simulink model "TORQUECONTROL"  (R2024b)
settings: Solver=FixedStepAuto  StartTime=0.0  StopTime=10.0  RelTol=1e-3  EnableMultiTasking=on
settings Model: DataDictionary=Master_Dictionary.sldd  EnableAccessToBaseWorkspace=off  Creator=torni  LastModifiedBy=Will
settings OptimizationCC: DefaultParameterBehavior=Inlined  EnhancedBackFolding=on  PassReuseOutputArgsAs=Individual arguments  ZeroExternalMemoryAtStartup=off  ZeroInternalMemoryAtStartup=off  MaxStackSize=8192  OptimizeBlockOrder=speed  DifferentSizesBufferReuse=on  OptimizationCustomize=off  EfficientTunableParamExpr=on
settings DebuggingCC: ParameterTunabilityLossMsg=error
settings HardwareCC: ProdBitPerPointer=32  ProdBitPerSizeT=32  ProdBitPerPtrDiffT=32  ProdLargestAtomicInteger=Long  ProdLargestAtomicFloat=Double  ProdWordSize=32  ProdLongLongMode=on  ProdHWDeviceType=ARM Compatible->ARM Cortex-M
settings SFSimCC: MATLABDynamicMemAlloc=off
settings RTWCC: Description=Embedded Coder  SystemTargetFile=ert.tlc  HardwareBoard=STM32H7xx Based (Single-core)  TemplateMakefile=ert_default_tmf  Toolchain=GNU Tools for ARM Embedded Processors
settings CodeAppCC: ForceParamTrailComments=on  IgnoreCustomStorageClasses=off  OperatorAnnotations=on  SimulinkDataObjDesc=on  SFDataObjDesc=on  InsertBlockDesc=on
settings ERTTargetCC: TargetLangStandard=C99 (ISO)  CodeReplacementLibrary=ARM Cortex-M  ExtModeTransport=3  ExtModeStaticAlloc=on  ExtModeStaticAllocSize=2048  ExtModeMexFile=ext_xcp  ExtModeIntrfLevel=Level2 - Open

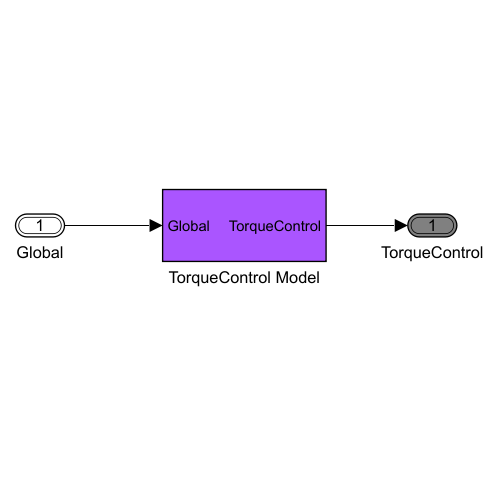
[thumbnail: Simulink's stored preview of the top-level diagram]
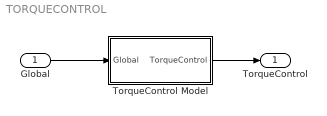
== system TORQUECONTROL ==
  "Global " : Inport  OutDataTypeStr=Bus: Global
  "TorqueControl Model " : Subsystem
  TorqueControl : Outport  OutDataTypeStr=Bus: TorqueControl  VectorParamsAs1DForOutWhenUnconnected=off
  wires:
  "Global "/1 -> "TorqueControl Model "/1(Global)
  "TorqueControl Model "/1(TorqueControl) -> TorqueControl/1

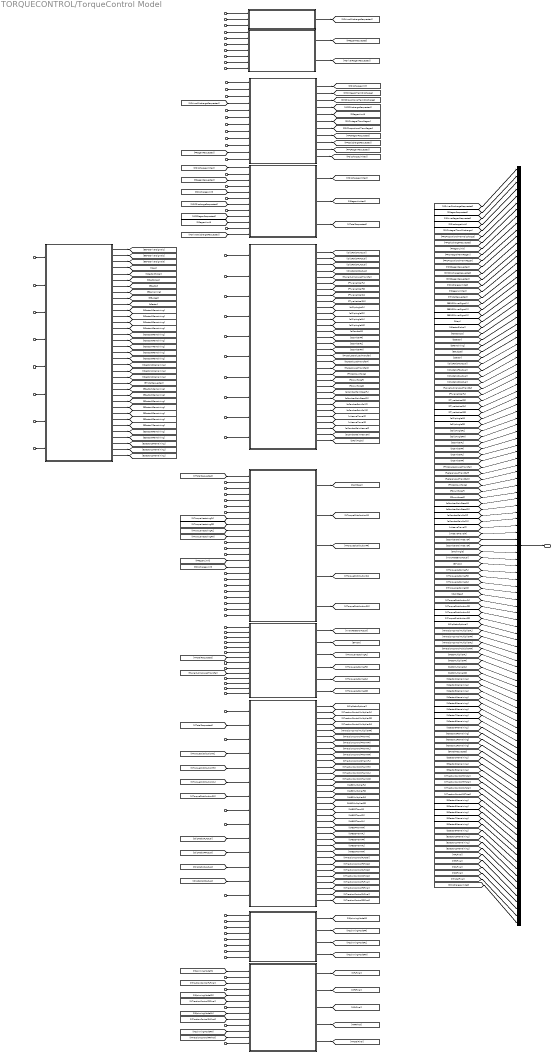
== system TORQUECONTROL/TorqueControl Model  ==
  note: Final output
  note: Distribution
  note: Energy & Vehicle State
  note: Total Torque Request
  note: Driver Requests
  note: Stages of Torque Control
      | 1. Driver Request
      | 2. Power Controller
      | 3. Total Torque Request
      | 4. Torque Distribution / Torque Vectoring
      | 5. Traction Control
      | 6. Spinning Mode Selection
  In Bus Element70 : Inport  PortName=Global  Element=InverterSignals.InverterRLSignals.nMotorRL
  In Bus Element74 : Inport  PortName=Global  Element=InverterSignals.InverterRLSignals.VDCInvRL
  In Bus Element : Inport  PortName=Global  Element=InverterSignals.InverterFLSignals.nMotorFL
  In Bus Element2 : Inport  PortName=Global  Element=InverterSignals.InverterRRSignals.nMotorRR
  In Bus Element3 : Inport  PortName=Global  Element=InverterSignals.InverterFRSignals.nMotorFR
  In Bus Element4 : Inport  PortName=Global  Element=Systems.pBrakeMax
  In Bus Element17 : Inport  PortName=Global  Element=Systems.pBrakeMax
  In Bus Element49 : Inport  PortName=Global  Element=Systems.pBrakeMax
  In Bus Element6 : Inport  PortName=Global  Element=Systems.BSpinningModeOn
  In Bus Element21 : Inport  PortName=Global  Element=Systems.BSpinningModeOn
  In Bus Element{7,16,37,48,57,62,79} (7 alike) : Inport  PortName=Global  Element=Systems.rThrottlePedal
  In Bus Element8 : Inport  PortName=Global  Element=Systems.NTCKdSelector
  In Bus Element{9,18,38..39,59,64,71,78} (8 alike) : Inport  PortName=Global  Element=Systems.vChassis
  In Bus Element10 : Inport  PortName=Global  Element=Systems.BTCOn
  In Bus Element11 : Inport  PortName=Global  Element=Systems.rGrip
  In Bus Element12 : Inport  PortName=Global  Element=Systems.rSteeringAngle
  In Bus Element14 : Inport  PortName=Global  Element=Systems.rTVMultiplier
  In Bus Element15 : Inport  PortName=Global  Element=Systems.BTVOn
  In Bus Element32 : Inport  PortName=Global  Element=Systems.BTVOn
  In Bus Element19 : Inport  PortName=Global  Element=Systems.aSteeringAngle
  In Bus Element1 : Inport  PortName=Global  Element=Systems.aSteeringAngle
  In Bus Element30 : Inport  PortName=Global  Element=Systems.rTorqueSplit
  In Bus Element31 : Inport  PortName=Global  Element=Systems.rEngineBrakingSplit
  In Bus Element33 : Inport  PortName=Global  Element=Systems.PEngineBraking
  In Bus Element34 : Inport  PortName=Global  Element=Systems.BInverterErrorFront
  In Bus Element35 : Inport  PortName=Global  Element=Systems.BInverterErrorRear
  In Bus Element{36,50,53,60,75} (5 alike) : Inport  PortName=Global  Element=Systems.rRegenPaddle
  In Bus Element51 : Inport  PortName=Global  Element=Systems.PActual
  In Bus Element58 : Inport  PortName=Global  Element=Systems.PActual
  In Bus Element63 : Inport  PortName=Global  Element=Systems.PActual
  In Bus Element52 : Inport  PortName=Global  Element=Systems.BEMSOn
  In Bus Element54 : Inport  PortName=Global  Element=Systems.sChassis
  In Bus Element55 : Inport  PortName=Global  Element=Systems.EOffset
  In Bus Element56 : Inport  PortName=Global  Element=Systems.rSOE
  In Bus Element67 : Inport  PortName=Global  Element=Systems.PRegenMax
  In Bus Element61 : Inport  PortName=Global  Element=Systems.PRegenMax
  In Bus Element68 : Inport  PortName=Global  Element=Systems.PDischargeMax
  In Bus Element69 : Inport  PortName=Global  Element=Systems.NPCKpSelector
  In Bus Element76 : Inport  PortName=Global  Element=Systems.MRegenMax
  In Bus Element77 : Inport  PortName=Global  Element=Systems.NThrottleMap
  In Bus Element81 : Inport  PortName=Global  Element=Systems.MMotorMaxFL
  In Bus Element86 : Inport  PortName=Global  Element=Systems.MMotorMaxFL
  In Bus Element83 : Inport  PortName=Global  Element=Systems.MMotorMaxFR
  In Bus Element87 : Inport  PortName=Global  Element=Systems.MMotorMaxFR
  In Bus Element84 : Inport  PortName=Global  Element=Systems.MMotorMaxRL
  In Bus Element88 : Inport  PortName=Global  Element=Systems.MMotorMaxRL
  In Bus Element85 : Inport  PortName=Global  Element=Systems.MMotorMaxRR
  In Bus Element89 : Inport  PortName=Global  Element=Systems.MMotorMaxRR
  In Bus Element5 : Inport  PortName=Global  Element=Stateflow.BReadyToDrive
  In Bus Element13 : Inport  PortName=Global  Element=GPSIMUSignals.nYawRateIMU
  In Bus Element40 : Inport  PortName=Global  Element=GPSIMUSignals.nYawRateIMU
  In Bus Element20 : Inport  PortName=Global  Element=GPSIMUSignals.gLongitudinalIMU
  In Bus Element42 : Inport  PortName=Global  Element=GPSIMUSignals.gLongitudinalIMU
  In Bus Element43 : Inport  PortName=Global  Element=GPSIMUSignals.gLateralIMU
  In Bus Element41 : Inport  PortName=Global  Element=GPSIMUSignals.vLateralIMU
  In Bus Element22 : Inport  PortName=Global  Element=Limitations.rSpeedRegenDerateFL
  In Bus Element23 : Inport  PortName=Global  Element=Limitations.rSpeedRegenDerateFR
  In Bus Element24 : Inport  PortName=Global  Element=Limitations.rSpeedRegenDerateRL
  In Bus Element25 : Inport  PortName=Global  Element=Limitations.rSpeedRegenDerateRR
  In Bus Element26 : Inport  PortName=Global  Element=Limitations.PTSTemperatureDerateRR
  In Bus Element27 : Inport  PortName=Global  Element=Limitations.PTSTemperatureDerateRL
  In Bus Element28 : Inport  PortName=Global  Element=Limitations.PTSTemperatureDerateFR
  In Bus Element29 : Inport  PortName=Global  Element=Limitations.PTSTemperatureDerateFL
  In Bus Element65 : Inport  PortName=Global  Element=Limitations.PRegenDerate
  In Bus Element80 : Inport  PortName=Global  Element=Limitations.PRegenDerate
  In Bus Element66 : Inport  PortName=Global  Element=Limitations.PDischargeDerate
  In Bus Element72 : Inport  PortName=Global  Element=Limitations.BDischargeAllowed
  In Bus Element82 : Inport  PortName=Global  Element=Limitations.BDischargeAllowed
  In Bus Element44 : Inport  PortName=Global  Element=WheelSpeeds.vWheelRR
  In Bus Element45 : Inport  PortName=Global  Element=WheelSpeeds.vWheelRL
  In Bus Element46 : Inport  PortName=Global  Element=WheelSpeeds.vWheelFR
  In Bus Element47 : Inport  PortName=Global  Element=WheelSpeeds.vWheelFL
  In Bus Element73 : Inport  PortName=Global  Element=BMSSignals.IIVTS
  Bus Creator1 : BusCreator  Inputs=113  OutDataTypeStr=Bus: TorqueControl
  Model : ModelReference  ModelNameDialog=MDriverRegenRequested.slx  SimulationMode=Normal  ModelReferenceVersion=13.6
  Model1 : ModelReference  ModelNameDialog=StateEstimation.slx  SimulationMode=Normal  ModelReferenceVersion=13.6
  Model10 : ModelReference  ModelNameDialog=MFinal.slx  SimulationMode=Normal  ModelReferenceVersion=13.6
  Model2 : ModelReference  ModelNameDialog=MDriverDischargeRequested.slx  SimulationMode=Normal  ModelReferenceVersion=13.6
  Model3 : ModelReference  ModelNameDialog=PowerController.slx  SimulationMode=Normal  ModelReferenceVersion=13.6
  Model4 : ModelReference  ModelNameDialog=MTotalRequested.slx  SimulationMode=Normal  ModelReferenceVersion=13.6
  Model5 : ModelReference  ModelNameDialog=EMS.slx  SimulationMode=Normal  ModelReferenceVersion=13.6
  Model6 : ModelReference  ModelNameDialog=TorqueVectoring.slx  SimulationMode=Normal  ModelReferenceVersion=13.6
  Model7 : ModelReference  ModelNameDialog=TorqueDistribution.slx  SimulationMode=Normal  ModelReferenceVersion=13.6
  Model8 : ModelReference  ModelNameDialog=TractionControl.slx  SimulationMode=Normal  ModelReferenceVersion=13.6
  Model9 : ModelReference  ModelNameDialog=SpinningMode.slx  SimulationMode=Normal  ModelReferenceVersion=13.6
  TorqueControl : Outport  OutDataTypeStr=Bus: TorqueControl  VectorParamsAs1DForOutWhenUnconnected=off
  wires:
  Model7/1 -> [rSplitRear]
  Model7/2 -> [MTorqueDistributionFL]
  Model7/3 -> [MTorqueDistributionFR]
  Model7/4 -> [MTorqueDistributionRL]
  Model7/5 -> [MTorqueDistributionRR]
  Model9/1 -> [MSpinningModeFL]
  Model9/2 -> [MSpinningModeFR]
  Model9/3 -> [MSpinningModeRL]
  Model9/4 -> [MSpinningModeRR]
  Bus Creator1/1 -> TorqueControl/1
  [MDriverDischargeRequested] -> Bus Creator1/1  "MDriverDischargeRequested"
  [MDriverRegenRequested] -> Bus Creator1/3  "MDriverRegenRequested"
  [MTotalRequested] -> Model7/1
  Model4/1 -> [MDischargeLimited]
  Model4/2 -> [MRegenLimited]
  Model4/3 -> [MTotalRequested]
  [PDischargeLimit] -> Model4/5
  [PRegenRequested] -> Model4/3
  [PDischargeLimited] -> Model4/1
  [MDischargeLimited] -> Bus Creator1/14  "MDischargeLimited"
  [MRegenLimited] -> Bus Creator1/15  "MRegenLimited"
  Model1/1 -> [rSlipRatioFLActual]
  Model1/2 -> [rSlipRatioFRActual]
  Model1/3 -> [rSlipRatioRLActual]
  Model1/4 -> [rSlipRatioRRActual]
  Model1/5 -> [FLongitudinalLoadTransfer]
  Model1/6 -> [FTyreVerticalFL]
  Model1/7 -> [FTyreVerticalFR]
  Model1/8 -> [FTyreVerticalRL]
  Model1/9 -> [FTyreVerticalRR]
  Model1/10 -> [aSlipAngleFL]
  Model1/11 -> [aSlipAngleFR]
  Model1/12 -> [aSlipAngleRL]
  Model1/13 -> [aSlipAngleRR]
  Model1/14 -> [aCamberFL]
  Model1/15 -> [aCamberFR]
  Model1/16 -> [aCamberRL]
  Model1/17 -> [aCamberRR]
  Model1/18 -> [FTotalLateralLoadTransfer]
  Model1/19 -> [FLateralLoadTransferF]
  Model1/20 -> [FLateralLoadTransferR]
  Model1/21 -> [FTotalDownforce]
  Model1/22 -> [FDownforceF]
  Model1/23 -> [FDownforceR]
  Model1/24 -> [aCamberGainSteerFL]
  Model1/25 -> [aCamberGainSteerFR]
  Model1/26 -> [aCamberGainRollF]
  Model1/27 -> [aCamberGainRollR]
  Model1/28 -> [xHeaveTravelF]
  Model1/29 -> [xHeaveTravelR]
  Model1/30 -> [aCamberGainHeaveF]
  Model1/31 -> [aCamberGainHeaveR]
  Model1/32 -> [aRollAngle]
  In Bus Element39/1 -> Model1/1
  In Bus Element47/1 -> Model1/2
  Model2/1 -> [MDriverDischargeRequested]
  Model10/1 -> [MFLFinal]
  Model10/2 -> [MFRFinal]
  Model10/3 -> [MRLFinal]
  Model10/4 -> [MRRFinal]
  Model10/5 -> [MTotalFinal]
  [MTractionControlFLFinal] -> Model10/3
  [MTractionControlFRFinal] -> Model10/6
  [MTractionControlRLFinal] -> Model10/9
  [MSpinningModeFL] -> Model10/1
  [MSpinningModeFR] -> Model10/5
  [MSpinningModeRL] -> Model10/8
  [MTorqueDistributionFL] -> Model8/4
  [MTorqueDistributionFR] -> Model8/5
  [MTorqueDistributionRL] -> Model8/6
  [MTorqueDistributionRR] -> Model8/7
  Model8/33 -> [MTractionControlRRFinal]
  Model8/32 -> [MTractionControlRLFinal]
  Model8/31 -> [MTractionControlFRFinal]
  Model8/30 -> [MTractionControlFLFinal]
  Model8/29 -> [MTractionControlRRTotal]
  Model8/28 -> [MTractionControlRLTotal]
  Model8/27 -> [MTractionControlFRTotal]
  Model8/26 -> [MTractionControlFLTotal]
  Model8/14 -> [NABSMultiplierFL]
  Model8/15 -> [NABSMultiplierFR]
  Model8/16 -> [NABSMultiplierRL]
  Model8/17 -> [NABSMultiplierRR]
  [MTotalRequested] -> Model8/2
  Model8/1 -> [rSlipRatioOptimal]
  Model8/2 -> [NTractionControlMultiplierFL]
  Model8/3 -> [NTractionControlMultiplierFR]
  Model8/4 -> [NTractionControlMultiplierRL]
  Model8/5 -> [NTractionControlMultiplierRR]
  Model8/6 -> [NTractionControlPTermFL]
  Model8/7 -> [NTractionControlPTermFR]
  Model8/8 -> [NTractionControlPTermRL]
  Model8/9 -> [NTractionControlPTermRR]
  Model8/13 -> [NTractionControlDTermRR]
  Model8/12 -> [NTractionControlDTermRL]
  Model8/10 -> [NTractionControlDTermFL]
  Model8/11 -> [NTractionControlDTermFR]
  Model8/18 -> [NABSPTermFL]
  Model8/19 -> [NABSPTermFR]
  Model8/20 -> [NABSPTermRL]
  Model8/21 -> [NABSPTermRR]
  Model8/22 -> [NABSDTermFL]
  Model8/23 -> [NABSDTermFR]
  Model8/24 -> [NABSDTermRL]
  Model8/25 -> [NABSDTermRR]
  [MDriverDischargeRequested] -> Model3/4
  Model/1 -> [PRegenRequested]
  [PRegenRequested] -> Bus Creator1/2  "PRegenRequested"
  [MTorqueVectoringFL] -> Model7/8
  [MTorqueVectoringRR] -> Model7/11
  [MTorqueVectoringRL] -> Model7/10
  [MTorqueVectoringFR] -> Model7/9
  Model5/1 -> [BEMSDriverSignal1]
  Model5/2 -> [BEMSDriverSignal2]
  Model5/4 -> [NLap]
  Model5/3 -> [BEMSDriverSignal3]
  Model3/10 -> [PPCRegenRequested]
  Model3/9 -> [PPCDischargeRequested]
  Model3/8 -> [MPCRegenRequested]
  Model3/7 -> [PPCProportionalTermRegen]
  Model3/6 -> [PPCIntegralTermRegen]
  Model3/5 -> [PRegenLimit]
  Model3/4 -> [MPCDischargeRequested]
  Model3/3 -> [PPCProportionalTermDischarge]
  Model3/2 -> [PPCIntegralTermDischarge]
  Model3/1 -> [PDischargeLimit]
  [PDischargeLimit] -> Bus Creator1/4  "PDischargeLimit"
  [PPCIntegralTermDischarge] -> Bus Creator1/5  "PPCIntegralTermDischarge"
  [PPCProportionalTermDischarge] -> Bus Creator1/6  "PPCProportionalTermDischarge"
  [MPCDischargeRequested] -> Bus Creator1/7  "MPCDischargeRequested"
  [PRegenLimit] -> Bus Creator1/8  "PRegenLimit"
  [PPCIntegralTermRegen] -> Bus Creator1/9  "PPCIntegralTermRegen"
  [PPCProportionalTermRegen] -> Bus Creator1/10  "PPCProportionalTermRegen"
  [MPCRegenRequested] -> Bus Creator1/11  "MPCRegenRequested"
  [PPCDischargeRequested] -> Bus Creator1/12  "PPCDischargeRequested"
  [PPCRegenRequested] -> Bus Creator1/13  "PPCRegenRequested"
  [PRegenRequested] -> Model3/11
  Model3/11 -> [PDischargeLimited]
  Model5/5 -> [NSectorGlobal]
  Model5/6 -> [NSectorLap]
  Model5/7 -> [ESector]
  Model5/8 -> [ERemaining]
  Model5/9 -> [EBudget]
  Model5/10 -> [sSector]
  In Bus Element73/1 -> Model/6
  [MPCDischargeRequested] -> Model4/7
  [PRegenLimit] -> Model4/10
  [MPCRegenRequested] -> Model4/9
  Model/2 -> [MDriverRegenRequested]
  Model6/6 -> [MTorqueVectoringRR]
  Model6/5 -> [MTorqueVectoringRL]
  Model6/4 -> [MTorqueVectoringFR]
  Model6/3 -> [MTorqueVectoringFL]
  Model6/2 -> [BTVOK]
  Model6/1 -> [nYawRateErrorActual]
  Model5/11 -> [NSector1Remaining]
  Model5/12 -> [NSector2Remaining]
  Model5/13 -> [NSector3Remaining]
  Model5/14 -> [NSector4Remaining]
  Model5/15 -> [NSector5Remaining]
  Model5/16 -> [NSector6Remaining]
  Model5/17 -> [NSector7Remaining]
  Model5/18 -> [NSector8Remaining]
  Model5/19 -> [NSector9Remaining]
  Model5/20 -> [NSector10Remaining]
  Model5/21 -> [NSector11Remaining]
  Model5/22 -> [NSector12Remaining]
  Model5/23 -> [ETotalRequested]
  Model5/24 -> [ESector1Remaining]
  Model5/25 -> [ESector2Remaining]
  Model5/26 -> [ESector3Remaining]
  Model5/27 -> [ESector4Remaining]
  Model5/28 -> [ESector5Remaining]
  Model5/29 -> [ESector6Remaining]
  Model5/30 -> [ESector7Remaining]
  Model5/31 -> [ESector8Remaining]
  Model5/32 -> [ESector9Remaining]
  Model5/33 -> [ESector10Remaining]
  Model5/34 -> [ESector11Remaining]
  Model5/35 -> [ESector12Remaining]
  [PDischargeLimit] -> Model7/16
  [PRegenLimit] -> Model7/15
  [MTotalRequested] -> Model6/7
  [FLongitudinalLoadTransfer] -> Model6/10
  [MSpinningModeRR] -> Model10/11
  [MTractionControlRRFinal] -> Model10/12
  [MTotalRequested] -> Bus Creator1/16  "MTotalRequested"
  [BEMSDriverSignal1] -> Bus Creator1/17  "BEMSDriverSignal1"
  [BEMSDriverSignal2] -> Bus Creator1/18  "BEMSDriverSignal2"
  [BEMSDriverSignal3] -> Bus Creator1/19  "BEMSDriverSignal3"
  [NLap] -> Bus Creator1/20  "NLap"
  [NSectorGlobal] -> Bus Creator1/21  "NSectorGlobal"
  [NSectorLap] -> Bus Creator1/22  "NSectorLap"
  [ESector] -> Bus Creator1/23  "ESector"
  [MTotalFinal] -> Bus Creator1/112  "MTotalFinal"
  [MRRFinal] -> Bus Creator1/111  "MRRFinal"
  [MRLFinal] -> Bus Creator1/110  "MRLFinal"
  [MFRFinal] -> Bus Creator1/109  "MFRFinal"
  [MFLFinal] -> Bus Creator1/108  "MFLFinal"
  [ESector12Remaining] -> Bus Creator1/107  "ESector12Remaining"
  [ESector11Remaining] -> Bus Creator1/106  "ESector11Remaining"
  [ESector10Remaining] -> Bus Creator1/105  "ESector10Remaining"
  [ESector9Remaining] -> Bus Creator1/104  "ESector9Remaining"
  [ESector8Remaining] -> Bus Creator1/103  "ESector8Remaining"
  [ESector7Remaining] -> Bus Creator1/102  "ESector7Remaining"
  [ESector6Remaining] -> Bus Creator1/101  "ESector6Remaining"
  [ESector5Remaining] -> Bus Creator1/100  "ESector5Remaining"
  [ESector4Remaining] -> Bus Creator1/99  "ESector4Remaining"
  [MTractionControlRRTotal] -> Bus Creator1/98  "MTractionControlRRTotal"
  [MTractionControlRLTotal] -> Bus Creator1/97  "MTractionControlRLTotal"
  [MTractionControlFRTotal] -> Bus Creator1/96  "MTractionControlFRTotal"
  [MTractionControlFLTotal] -> Bus Creator1/95  "MTractionControlFLTotal"
  [ESector3Remaining] -> Bus Creator1/94  "ESector3Remaining"
  [ESector2Remaining] -> Bus Creator1/93  "ESector2Remaining"
  [ESector1Remaining] -> Bus Creator1/92  "ESector1Remaining"
  [ETotalRequested] -> Bus Creator1/91  "ETotalRequested"
  [NSector12Remaining] -> Bus Creator1/90  "NSector12Remaining"
  [NSector11Remaining] -> Bus Creator1/89  "NSector11Remaining"
  [NSector10Remaining] -> Bus Creator1/88  "NSector10Remaining"
  [NSector9Remaining] -> Bus Creator1/87  "NSector9Remaining"
  [NSector8Remaining] -> Bus Creator1/86  "NSector8Remaining"
  [NSector7Remaining] -> Bus Creator1/85  "NSector7Remaining"
  [NSector6Remaining] -> Bus Creator1/84  "NSector6Remaining"
  [NSector5Remaining] -> Bus Creator1/83  "NSector5Remaining"
  [NSector4Remaining] -> Bus Creator1/82  "NSector4Remaining"
  [NSector3Remaining] -> Bus Creator1/81  "NSector3Remaining"
  [NSector2Remaining] -> Bus Creator1/80  "NSector2Remaining"
  [NSector1Remaining] -> Bus Creator1/79  "NSector1Remaining"
  [NABSMultiplierRR] -> Bus Creator1/78  "NABSMultiplierRR"
  [NABSMultiplierRL] -> Bus Creator1/77  "NABSMultiplierRL"
  [NABSMultiplierFR] -> Bus Creator1/76  "NABSMultiplierFR"
  [NABSMultiplierFL] -> Bus Creator1/75  "NABSMultiplierFL"
  [NTractionControlMultiplierRR] -> Bus Creator1/74  "NTractionControlMultiplierRR"
  [NTractionControlMultiplierRL] -> Bus Creator1/73  "NTractionControlMultiplierRL"
  [NTractionControlMultiplierFR] -> Bus Creator1/72  "NTractionControlMultiplierFR"
  [NTractionControlMultiplierFL] -> Bus Creator1/71  "NTractionControlMultiplierFL"
  [rSlipRatioOptimal] -> Bus Creator1/70  "rSlipRatioOptimal"
  [MTorqueDistributionRR] -> Bus Creator1/69  "MTorqueDistributionRR"
  [MTorqueDistributionRL] -> Bus Creator1/68  "MTorqueDistributionRL"
  [MTorqueDistributionFR] -> Bus Creator1/67  "MTorqueDistributionFR"
  [MTorqueDistributionFL] -> Bus Creator1/66  "MTorqueDistributionFL"
  [MTorqueVectoringRR] -> Bus Creator1/64  "MTorqueVectoringRR"
  [rSplitRear] -> Bus Creator1/65  "rSplitRear"
  [MTorqueVectoringRL] -> Bus Creator1/63  "MTorqueVectoringRL"
  [MTorqueVectoringFR] -> Bus Creator1/62  "MTorqueVectoringFR"
  [MTorqueVectoringFL] -> Bus Creator1/61  "MTorqueVectoringFL"
  [nYawRateErrorActual] -> Bus Creator1/59  "nYawRateErrorActual"
  [aRollAngle] -> Bus Creator1/58  "aRollAngle"
  [aCamberGainHeaveR] -> Bus Creator1/57  "aCamberGainHeaveR"
  [aCamberGainHeaveF] -> Bus Creator1/56  "aCamberGainHeaveF"
  [xHeaveTravelR] -> Bus Creator1/55  "xHeaveTravelR"
  [xHeaveTravelF] -> Bus Creator1/54  "xHeaveTravelF"
  [aCamberGainRollR] -> Bus Creator1/53  "aCamberGainRollR"
  [aCamberGainRollF] -> Bus Creator1/52  "aCamberGainRollF"
  [aCamberGainSteerFR] -> Bus Creator1/51  "aCamberGainSteerFR"
  [aCamberGainSteerFL] -> Bus Creator1/50  "aCamberGainSteerFL"
  [FDownforceR] -> Bus Creator1/49  "FDownforceR"
  [FDownforceF] -> Bus Creator1/48  "FDownforceF"
  [FTotalDownforce] -> Bus Creator1/47  "FTotalDownforce"
  [FLateralLoadTransferR] -> Bus Creator1/46  "FLateralLoadTransferR"
  [FLateralLoadTransferF] -> Bus Creator1/45  "FLateralLoadTransferF"
  [FTotalLateralLoadTransfer] -> Bus Creator1/44  "FTotalLateralLoadTransfer"
  [aCamberRR] -> Bus Creator1/43  "aCamberRR"
  [aCamberRL] -> Bus Creator1/42  "aCamberRL"
  [aCamberFR] -> Bus Creator1/41  "aCamberFR"
  [aCamberFL] -> Bus Creator1/40  "aCamberFL"
  [aSlipAngleRR] -> Bus Creator1/39  "aSlipAngleRR"
  [aSlipAngleRL] -> Bus Creator1/38  "aSlipAngleRL"
  [aSlipAngleFR] -> Bus Creator1/37  "aSlipAngleFR"
  [aSlipAngleFL] -> Bus Creator1/36  "aSlipAngleFL"
  [FTyreVerticalRR] -> Bus Creator1/35  "FTyreVerticalRR"
  [FTyreVerticalRL] -> Bus Creator1/34  "FTyreVerticalRL"
  [FTyreVerticalFR] -> Bus Creator1/33  "FTyreVerticalFR"
  [FTyreVerticalFL] -> Bus Creator1/32  "FTyreVerticalFL"
  [FLongitudinalLoadTransfer] -> Bus Creator1/31  "FLongitudinalLoadTransfer"
  [rSlipRatioRRActual] -> Bus Creator1/30  "rSlipRatioRRActual"
  [ERemaining] -> Bus Creator1/24  "ERemaining"
  [EBudget] -> Bus Creator1/25  "EBudget"
  [sSector] -> Bus Creator1/26  "sSector"
  [rSlipRatioFLActual] -> Bus Creator1/27  "rSlipRatioFLActual"
  [rSlipRatioFRActual] -> Bus Creator1/28  "rSlipRatioFRActual"
  [rSlipRatioRLActual] -> Bus Creator1/29  "rSlipRatioRLActual"
  In Bus Element78/1 -> Model2/2
  In Bus Element79/1 -> Model2/3
  In Bus Element76/1 -> Model/1
  In Bus Element75/1 -> Model/2
  In Bus Element64/1 -> Model/3
  In Bus Element74/1 -> Model/5
  In Bus Element71/1 -> Model3/1
  In Bus Element69/1 -> Model3/2
  In Bus Element68/1 -> Model3/3
  In Bus Element60/1 -> Model3/10
  In Bus Element62/1 -> Model3/9
  In Bus Element63/1 -> Model3/8
  In Bus Element65/1 -> Model3/7
  In Bus Element66/1 -> Model3/6
  In Bus Element67/1 -> Model3/5
  In Bus Element50/1 -> Model4/8
  In Bus Element57/1 -> Model4/6
  In Bus Element58/1 -> Model4/4
  In Bus Element59/1 -> Model4/2
  In Bus Element56/1 -> Model5/8
  In Bus Element55/1 -> Model5/7
  In Bus Element54/1 -> Model5/6
  In Bus Element53/1 -> Model5/5
  In Bus Element52/1 -> Model5/4
  In Bus Element51/1 -> Model5/3
  In Bus Element49/1 -> Model5/2
  In Bus Element48/1 -> Model5/1
  In Bus Element44/1 -> Model1/5
  In Bus Element45/1 -> Model1/4
  In Bus Element46/1 -> Model1/3
  In Bus Element43/1 -> Model1/6
  In Bus Element42/1 -> Model1/7
  In Bus Element1/1 -> Model1/10
  In Bus Element40/1 -> Model1/9
  In Bus Element38/1 -> Model7/2
  In Bus Element18/1 -> Model6/3
  In Bus Element9/1 -> Model8/9
  In Bus Element37/1 -> Model7/3
  In Bus Element35/1 -> Model7/5
  In Bus Element34/1 -> Model7/6
  In Bus Element33/1 -> Model7/7
  In Bus Element32/1 -> Model7/12
  In Bus Element31/1 -> Model7/13
  In Bus Element30/1 -> Model7/14
  In Bus Element29/1 -> Model7/17
  In Bus Element28/1 -> Model7/18
  In Bus Element27/1 -> Model7/19
  In Bus Element26/1 -> Model7/20
  In Bus Element36/1 -> Model7/4
  In Bus Element20/1 -> Model6/1
  In Bus Element19/1 -> Model6/2
  In Bus Element17/1 -> Model6/4
  In Bus Element16/1 -> Model6/5
  In Bus Element15/1 -> Model6/6
  In Bus Element14/1 -> Model6/8
  In Bus Element13/1 -> Model6/9
  In Bus Element12/1 -> Model8/1
  In Bus Element11/1 -> Model8/3
  In Bus Element10/1 -> Model8/8
  [rSlipRatioFLActual] -> Model8/10
  [rSlipRatioFRActual] -> Model8/11
  [rSlipRatioRLActual] -> Model8/12
  [rSlipRatioRRActual] -> Model8/13
  In Bus Element8/1 -> Model8/14
  In Bus Element6/1 -> Model9/2
  In Bus Element/1 -> Model9/6
  In Bus Element3/1 -> Model9/7
  In Bus Element2/1 -> Model9/8
  In Bus Element4/1 -> Model9/4
  In Bus Element5/1 -> Model9/3
  In Bus Element7/1 -> Model9/1
  In Bus Element25/1 -> Model10/13
  In Bus Element24/1 -> Model10/10
  In Bus Element23/1 -> Model10/7
  In Bus Element22/1 -> Model10/4
  In Bus Element21/1 -> Model10/2
  [BTVOK] -> Bus Creator1/60  "BTVOK"
  In Bus Element70/1 -> Model9/5
  In Bus Element77/1 -> Model2/1
  In Bus Element72/1 -> Model3/12
  In Bus Element61/1 -> Model/4
  In Bus Element80/1 -> Model/7
  [PDischargeLimited] -> Bus Creator1/113  "PDischargeLimited"
  In Bus Element82/1 -> Model4/11
  [MDriverDischargeRequested] -> Model4/12
  In Bus Element41/1 -> Model1/8
  In Bus Element85/1 -> Model7/23
  In Bus Element84/1 -> Model7/24
  In Bus Element81/1 -> Model7/22
  In Bus Element83/1 -> Model7/21
  In Bus Element87/1 -> Model6/12
  In Bus Element86/1 -> Model6/11
  In Bus Element88/1 -> Model6/13
  In Bus Element89/1 -> Model6/14
